simulink model "eTimer_QD"  (Simulink 8.1)
settings: Solver=FixedStepDiscrete  StartTime=0.0  StopTime=10.0  FixedStep=0.2  RelTol=1e-3
undefined symbols (not defined in the file or in its folder): A14, B, B13, D, L3, PD10, PD11, R10, R16, T15
libraries: rappid_564xl_ec_toolbox x8
settings Model: Creator=evarshavskaya  LastModifiedBy=evarshavskaya
settings DataIOCC: ExternalInput=off  InitialState=off  SaveOutput=off  SignalLogging=off  SaveTime=off
settings OptimizationCC: InlineParams=on  OptimizeModelRefInitCode=on  LifeSpan=1
settings DebuggingCC: InheritedTsInSrcMsg=none  SingleTaskRateTransMsg=error  UnconnectedInputMsg=error  UnconnectedOutputMsg=error  UnconnectedLineMsg=error  UnknownTsInhSupMsg=error
settings HardwareCC: ProdLargestAtomicInteger=Long  ProdLargestAtomicFloat=Double  ProdIntDivRoundTo=Zero  ProdEndianess=BigEndian  ProdHWDeviceType=Freescale->32-bit PowerPC
settings RTWCC: SystemTargetFile=rappid564xl.tlc  MakeCommand=rappid_564xl_make_rtw  TemplateMakefile=rappid_564xl_default_tmf  PostCodeGenCommand=rappid_analyzegencode(buildInfo)  Description=RAppID Toolbox MPC564xL Code Generation Target (rappid)  ProcessScript=rappid564xl_make_rtw_hook
settings CodeAppCC: IgnoreCustomStorageClasses=off  CustomSymbolStrType=$N$R$M  InternalIdentifier=Classic
settings STFCustomTargetCC: CodeReplacementLibrary=ANSI_C  ModelReferenceCompliant=off  CombineOutputUpdateFcns=on  SuppressErrorStatus=on  ERTCustomFileBanners=on  SupportContinuousTime=off  SupportNonInlinedSFcns=off  MATLABClassNameForMDSCustomization=Simulink.SoftwareTarget.ERTCustomization  GRTInterface=off  SystemTargetFile=rappid564xl.tlc
settings ERTTargetCC: CodeReplacementLibrary=ANSI_C  MultiwordLength=2048  ModelReferenceCompliant=off  ParMdlRefBuildCompliant=off  CompOptLevelCompliant=off  ConcurrentExecutionCompliant=off  SuppressErrorStatus=on  ERTFirstTimeCompliant=off  ModelStepFunctionPrototypeControlCompliant=off  CPPClassGenCompliant=off  InlinedParameterPlacement=NonHierarchical  ERTCustomFileTemplate=example_file_process.tlc  ConvertIfToSwitch=off  SuppressUnreachableDefaultCases=off

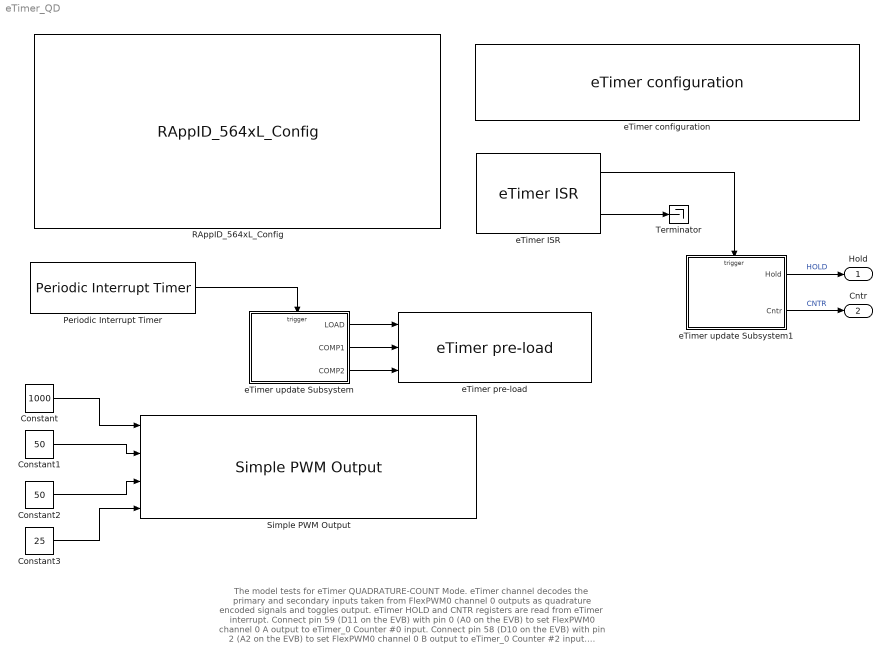
== system eTimer_QD ==
  note: The model tests for eTimer QUADRATURE-COUNT Mode.
      |
      | eTimer channel decodes the primary and secondary inputs taken from FlexPWM0 channel 0 outputs as quadrature encoded
      | signals and toggles output. eTimer HOLD and CNTR registers are read from eTimer interrupt.
      |
      | Connect pin 59 (D11 on the EVB) with pin 0 (A0 on the EVB) to set FlexPWM0 channel 0 A output to eTimer_0 Counter #0 input.
      | Connect pin 58 (D10 on the EVB) with pin 2 (A2 on the EVB) to set FlexPWM0 channel 0 B output to eTimer_0 Counter #2 input.
      |
      | Connect pin 58 (D10 on the EVB) to the scope to watch FlexPWM0 channel 0 A output
      | Connect pin 59 (D11 on the EVB) to the scope to watch FlexPWM0 channel 0 B output
      | Connect pin 1  (A1 on the EVB) to the scope to watch eTimer0 channel 1 output
  Constant : Constant  Value=1000  OutDataTypeStr=uint32
  Constant1 : Constant  Value=50  OutDataTypeStr=uint32
  Constant2 : Constant  Value=50  OutDataTypeStr=uint32
  Constant3 : Constant  Value=25  OutDataTypeStr=uint32
  Periodic Interrupt Timer : rappid_564xl_ec_toolbox/MPC564xL/General Purpose Blocks/Periodic Interrupt Timer  pit_chan=1  pit_timeout=200  int_priority=13  pit_timeout_val=23999999
  RAppID_564xL_Config : rappid_564xl_ec_toolbox/MPC564xL/RAppID_564xL_Config  SystemClock=120  XTAL=40  MC_clock_60=12  MC_clock_80=16  MC_clock_120=10  SWG_clock_60=20  SWG_clock_80=13.334  SWG_clock_120=20  Compiler=CodeWarrior  MemTarget=RAM  Part=MPC5643L  Package=144 LQFP  global_int_priority=10  base_tick_priority=14  sys_task_supress=off  exception_handlers=off  stored_mdl_name=eTimer_QD  freemaster_interface=Oops  freemaster_rx_pin="LINFlex_0 Rx Pin 116 : \"PB[3]\""  freemaster_tx_pin="LINFlex_0 Tx Pin 114 : \"PB[2]\""  freemaster_interface_1=Serial 0  freemaster_enable=on  freemaster_rate=57600  freemaster_tx0_pin=18 : B[2] : 114 : A14  freemaster_rx0_pin=19 : B[3] : 116 : B13  freemaster_tx1_pin=57 : D[9] : 26 : L3  freemaster_rx1_pin=29 : B[13] : 60 : R10  freemaster_can_channel=1CH  freemater_can_speed=500K  freemaster_can_msgig=0x7AA  ccp_interface=None  ccp_enable=off  ccp_can_channel=CH1 (MB 0 - 1)  ccp_can_speed=500K  ccp_can_cro_id=256  ccp_can_dto_id=257  ccp_dev_id=RappID  ccp_dev_addr=0  ccp_odt=3  ccp_daq=3  pil_enable=off  pil_bam=on  comport=1  pil_rate=57600  bam_password_def=on  bam_password=0xFEEDFACECAFEBEEF  bam_sa_cs=off  bam_start_address=0x0  bam_code_size=0x7000  cons_dspi=on  cons_can=on  cons_adc=on  cons_pwm=on  cons_ctu=on  cons_swg=on  cons_eTimer=on  cons_fm=on
  Simple PWM Output : rappid_564xl_ec_toolbox/MPC564xL/Motor Control Blocks/Simple PWM Output  pwmModule=0  pwmMod=0  SubModule=0  subMod=0  InitFreq=1000  resolution=1 %  resValue=1  InitDutyA=50  InitDutyB=50  align=A - edge aligned B - phase shifted  PhaseShift_A=0  PhaseShift=25  Phase_A=0  Phase_B=25  centered=-1  DoubleS=off  doubleSw=off  debugSw=off  debug_mode=0  pin_A0="58  : PD10 : [ 76 ] : [ T15 ]"  pin_B0="59  : PD11 : [ 78 ] : [ R16 ]"  pin_X0=None  pin_A1=None  pin_B1=None  pin_X1=None  pin_A2=None  pin_B2=None  pin_X2=None  pin_A3=None  pin_B3=None  pin_X3=None  pin1_A0=None  pin1_B0=None  pin1_X0=None  pin1_A1=None  pin1_B1=None  pin1_X1=None  pin1_A2=None  pin1_B2=None  pin1_X2=None  pin1_A3=None  pin1_B3=None  pin1_X3=None  pcrNumA=58  pcrNumB=59  pcrNumX=255  polA=off  polB=off  polX=off  octrl=0  syncFrom0=off  masterSync=0  outVal0=off  outVal1=off  outVal2=on  outVal3=on  outVal4=on  outVal5=on  outTrig=60
  Terminator : Terminator
  eTimer ISR : rappid_564xl_ec_toolbox/MPC564xL/Motor Control Blocks/eTimer ISR  SubModule=0  Timerchan=1  subMod=0  channel=1  isrPriority=14  isrPrio=14
  eTimer configuration : rappid_564xl_ec_toolbox/MPC564xL/Motor Control Blocks/eTimer configuration  SubModule=0  TimerChan=1  subMod=0  channel=1  CountMode=100 - Quadrature count mode using primary and secondary sources  CNTMODE=4  CountOnce=0 - Count repeatedly  ONCE=0  CountLength=1 - Count until compare and then reinitialize  LENGTH=1  CountDirection=0 - Count up  DIR=0  OutputEnable=1 - Output signal is driven to the external pin  OEN=1  CoChanInit=00 - Other channels cannot force re-initialization of this channel  COINIT=0  StopAction=0 - Output enable is unaffected by stop mode  STPEN=0  ReloadOnCapt=00 - Do not reload the counter on a capture event  ROC=0  PrimarySource=00010 - Counter #2 input pin  PRISRC=2  PrimSrcPol=0 - True polarity  PIPS=0  SecondarySource=00000 - Counter #0 input pin  SECSRC=0  SecSrcPol=0 - True polarity  SIPS=0  FILT_CNT=0  FILT_PER=0  FILT=0  OutputMode=0011 - Toggle output on successful compare (COMP1 or COMP2)  OUTMODE=3  OutputPol=0 - True polarity  OPS=0  MasterMode=0 - Disable broadcast of this channel output  MSTR=0  ForcedOutVal=0  VAL=0  CoForce=0 - Other channels cannot force this channel output  COFRC=0  CompLoad1=010 - Load COMP1 with CMPLD1 upon successful compare with the value in COMP1  CLC1=2  CompLoad2=101 - Load COMP2 with CMPLD2 upon successful compare with the value in COMP2  CLC2=5  CompareMode="00 - COMP1 and COMP2  are used when the counter is counting up"  CMPMODE=0  CaptMode1=10 - Capture rising edges  CPT1MODE=2  CaptMode2=00 - Capture disabled  CPT2MODE=0  OneShCaptMode=0 - Free running mode is selected  ONESHOT=0  CaptFIFO=0  CFWM=0  CNTRinit=1  COMP1init=10  COMP2init=10  mod0ch0pin="0   : PA0  : [ 73 ] : [ T14 ]  input/output"  mod0ch1pin="1   : PA1  : [ 74 ] : [ R14 ]  input/output"  mod0ch2pin="2   : PA2  : [ 84 ] : [ N16 ]  input/output"  mod0ch3pin=None  mod0ch4pin=None  mod0ch5pin=None  mod1ch0pin=None  mod1ch1pin=None  mod1ch2pin=None  mod1ch3pin=None  mod1ch4pin=None  mod1ch5pin=None  mod2ch0pin=None  mod2ch1pin=None  mod2ch2pin=None  mod2ch3pin=None  mod2ch4pin=None  mod2ch5pin=None  pcrNum0=0  pcrNum1=1  pcrNum2=2  pcrNum3=255  pcrNum4=255  pcrNum5=255  TCFIE=off  TCF1IE=off  TCF2IE=off  TOFIE=off  IELFIE=on  IEHFIE=on  ICF1IE=off  ICF2IE=off  INTDMA=48
  eTimer pre-load : rappid_564xl_ec_toolbox/MPC564xL/Motor Control Blocks/eTimer pre-load  SubModule=0  Timerchan=1  subMod=0  channel=1
  eTimer update Subsystem : Subsystem  TreatAsAtomicUnit=on
      settings: RTWSystemCode=Nonreusable function
  eTimer update Subsystem1 : Subsystem  TreatAsAtomicUnit=on
      settings: RTWSystemCode=Nonreusable function
  Hold : Outport
  Cntr : Outport  Port=2
  wires:
  Constant/1 -> Simple PWM Output/1
  Constant1/1 -> Simple PWM Output/2
  Periodic Interrupt Timer/1 -> eTimer update Subsystem/Trigger
  eTimer update Subsystem/1(LOAD) -> eTimer pre-load/1
  eTimer update Subsystem/2(COMP1) -> eTimer pre-load/2
  eTimer update Subsystem/3(COMP2) -> eTimer pre-load/3
  Constant2/1 -> Simple PWM Output/3
  Constant3/1 -> Simple PWM Output/4
  eTimer update Subsystem1/1(Hold) -> Hold/1  "HOLD"
  eTimer update Subsystem1/2(Cntr) -> Cntr/1  "CNTR"
  eTimer ISR/1 -> eTimer update Subsystem1/Trigger
  eTimer ISR/2 -> Terminator/1

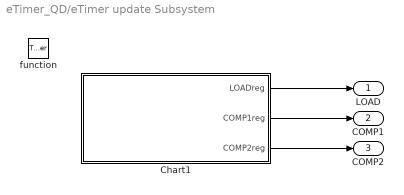
== system eTimer_QD/eTimer update Subsystem ==
  function : TriggerPort  TriggerType=function-call
  Chart1 : Stateflow chart  TreatAsAtomicUnit=on
  LOAD : Outport
  COMP1 : Outport  Port=2
  COMP2 : Outport  Port=3
  wires:
  Chart1/3(COMP2reg) -> COMP2/1
  Chart1/2(COMP1reg) -> COMP1/1
  Chart1/1(LOADreg) -> LOAD/1

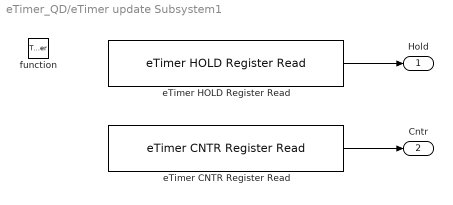
== system eTimer_QD/eTimer update Subsystem1 ==
  function : TriggerPort  TriggerType=function-call
  eTimer CNTR Register Read : rappid_564xl_ec_toolbox/MPC564xL/Motor Control Blocks/eTimer CNTR Register Read  SubModule=0  TimerChan=1  subMod=0  channel=1
  eTimer HOLD Register Read : rappid_564xl_ec_toolbox/MPC564xL/Motor Control Blocks/eTimer HOLD Register Read  SubModule=0  TimerChan=1  subMod=0  channel=1
  Hold : Outport
  Cntr : Outport  Port=2
  wires:
  eTimer HOLD Register Read/1 -> Hold/1
  eTimer CNTR Register Read/1 -> Cntr/1

== stateflow chart eTimer update Subsystem/Chart1 ==
  settings: executeAtInitialization=1
  state A
    du:
    LOADreg=1;
    COMP1reg=20;
    COMP2reg=20;
    int_counter=int_counter+1;
  state A1
    du:
    LOADreg=1;
    COMP1reg=10;
    COMP2reg=10;
    int_counter=int_counter-1;
  (default) -> A : {int_counter=0;}
  A1 -> A : [int_counter < 2]
  A -> A1 : [int_counter > 10]
  data: LOADreg output uint16; COMP1reg output uint16; int_counter local uint32 =0; COMP2reg output uint16
